simulink model "Adaptive_control_CSAD_model"  (R2017a)
settings: Solver=ode4  StartTime=0.0  StopTime=t_sim  FixedStep=0.01  RelTol=1e-3
values from neighbouring files (symbols this model uses):
  controller = 1    [Run4corner.m]
  eta_initial = [5; -1; 0]    [Run4corner.m]    (also in Simulation_plot.m = [-4; -2; 0.6*pi])
  gamma = 1.5    [Run4corner.m]
  mrs_select = 0    [Run4corner.m]
  nu_initial = [0; 0; 0]    [Run4corner.m]    (also in Simulation_plot.m)
  rho = 0.8    [Run4corner.m]
  sigma = 2    [Run4corner.m]
undefined symbols (not defined in the file or in its folder): fdesignblkfcn, gcbh
libraries: simulink x4, dsparch4 x1
(part 2 of 2)

== matlab function Adaptive_control_CSAD_model/L1 Cascade/Velocity Controller ==
  data: tau input; eta input; Alpha_DWC input; Alpha_DWC_dot input; Tau_c output; w_delta_hat_dot output; Nu input; model input; eta_hat_dot output; nu_hat_dot output; w_delta_hat input; eta_hat input; nu_hat input
function [Tau_c,w_delta_hat_dot,eta_hat_dot,nu_hat_dot]= VelocityControl(tau,eta,Alpha_DWC, Alpha_DWC_dot,Nu,model,w_delta_hat,eta_hat,nu_hat)

M = model(1:3,1:3);
C = model(1:3,4:6);
D = model(1:3,7:9);

z2 = Nu - Alpha_DWC;
psi=eta(3);
Gamma2 = diag([0.2,0.2 , 0.1745])*M;
delta_v = 0.7;
delta_r = 1;

z2_v = [z2(1), z2(2)]';
z2_r = z2(3);

first = 1/(sqrt(z2_v'*z2_v + delta_v^2));
second = 1/(sqrt(z2_r^2 + delta_r^2));

K2 = Gamma2*[first*eye(2,2) zeros(2,1); zeros(1,2) second];

z2 = Nu - Alpha_DWC;


R_T = [cos(psi) -sin(psi) 0;
       sin(psi) cos(psi) 0;
       0 0 1]';
eta_tilde = eta_hat - eta;
nu_tilde = nu_hat - Nu;


gamma_w_delta = (20*pi)^2/4; 
L1 = eye(3)*(2*pi)^2;
L2 = eye(3)*2*1.2*2*pi*3;

eta_hat_dot = -L1*eta_tilde + R_T'*Nu;
nu_hat_dot = -L2*nu_tilde + M\(tau+w_delta_hat-C*Nu-D*Nu);

w_delta_hat_dot=-gamma_w_delta*nu_tilde;

%linear model
Tau_c = M * Alpha_DWC_dot + C*Alpha_DWC+ D * Alpha_DWC - K2 * z2 -w_delta_hat;


end

== matlab function Adaptive_control_CSAD_model/L1 Cascade/ Pose Controller ==
  data: Eta_t input; Eta_tdot input; Eta_tddot input; Eta input; Nu input; Alpha output; Alphadot output
function [ Alpha ,Alphadot]  = PoseControl(Eta_t, Eta_tdot,Eta_tddot, Eta, Nu)
Gamma1 =  diag([0.08, 0.08, 0.0697]);
delta_psi = 0.5;
delta_p = 0.5;

psi = Eta(3);
r = Nu(3);

S = [0 -r  0; r  0  0; 0  0  0];
S_T = S';
R = [cos(psi) -sin(psi) 0; sin(psi) cos(psi) 0; 0 0 1];
R_T = R';

z1 = R_T * (Eta - Eta_t);

z1_p = [z1(1), z1(2)]';
z1_psi = z1(3);

first = 1/(sqrt(z1_p'*z1_p + delta_p^2));
second = 1/(sqrt(z1_psi^2 + delta_psi^2));

K1 = Gamma1*[first*eye(2,2) zeros(2,1); zeros(1,2) second];

Nu_d = R_T * Eta_tdot - K1 * z1;
Alpha = Nu_d;
z2 = Nu - Alpha;

z1dot = S_T * z1 - K1 * z1 + z2;

z1_p = [z1(1), z1(2)]';
z1_psi = z1(3);
z1_pdot = [z1dot(1), z1dot(2)]';
z1_psidot = z1dot(3);

first2 = (z1_p'*z1_pdot)/((z1_p'*z1_p + delta_p^2)^(3/2));

second2 = (z1_psi*z1_psidot)/((z1_psi^2 + delta_psi^2)^(3/2));

K1dot = - Gamma1*[first2*eye(2,2) zeros(2,1); zeros(1,2) second2];

Alphadot = R_T * Eta_tddot + S_T * R_T * Eta_tdot - K1dot * z1 - K1*z1dot;

end

== matlab function Adaptive_control_CSAD_model/Immersion and Invariance/ Pose Controller ==
  data: tau input; Eta_t input; Eta_tdot input; Eta_tddot input; Eta input; Nu input; model input; tau output; phi_dot_hat output; phi_hat input
function [tau,phi_dot_hat]  = Immersion(tau,Eta_t, Eta_tdot,Eta_tddot, Eta, Nu,model,phi_hat)

M = model(1:3,1:3);
C = model(1:3,4:6);
D = model(1:3,7:9);

Gamma1 =  diag([0.08, 0.08, 0.0697]);
delta_psi = 0.5;
delta_p = 0.5;

psi = Eta(3);
r = Nu(3);

S = [0 -r  0; r  0  0; 0  0  0];
S_T = S';
R = [cos(psi) -sin(psi) 0; sin(psi) cos(psi) 0; 0 0 1];
R_T = R';

z1 = R_T * (Eta - Eta_t);

z1_p = [z1(1), z1(2)]';
z1_psi = z1(3);

first = 1/(sqrt(z1_p'*z1_p + delta_p^2));
second = 1/(sqrt(z1_psi^2 + delta_psi^2));

K1 = Gamma1*[first*eye(2,2) zeros(2,1); zeros(1,2) second];

Nu_d = R_T * Eta_tdot - K1 * z1;
Alpha = Nu_d;
z2 = Nu - Alpha;

z1dot = S_T * z1 - K1 * z1 + z2;

z1_p = [z1(1), z1(2)]';
z1_psi = z1(3);
z1_pdot = [z1dot(1), z1dot(2)]';
z1_psidot = z1dot(3);

first2 = (z1_p'*z1_pdot)/((z1_p'*z1_p + delta_p^2)^(3/2));

second2 = (z1_psi*z1_psidot)/((z1_psi^2 + delta_psi^2)^(3/2));

K1dot = - Gamma1*[first2*eye(2,2) zeros(2,1); zeros(1,2) second2];

Alphadot = R_T * Eta_tddot + S_T * R_T * Eta_tdot - K1dot * z1 - K1*z1dot;


Gamma= diag([8, 4, 8, 8, 8, 4, 8, 8,0.4,0.4,0.4]);


r = Nu(3);
v=Nu(2);

z2 = Nu - Alpha;

Gamma2 = diag([0.2,0.2 , 0.1745])*M;
delta_v = 0.7;
delta_r = 1;

z2_v = [z2(1), z2(2)]';
z2_r = z2(3);

first = 1/(sqrt(z2_v'*z2_v + delta_v^2));
second = 1/(sqrt(z2_r^2 + delta_r^2));

K2 = Gamma2*[first*eye(2,2) zeros(2,1); zeros(1,2) second];


Phi = [0 0 0 0 0 0 0 0; abs(r)*v r abs(v)*r abs(r)*r 0 0 0 0; 0 0 0 0 abs(r)*v r abs(v)*r abs(r)*r];
Phi = [Phi R_T];
phi_dot_hat = -Gamma* Phi' * ( tau- C*Nu - D*Nu  +  Phi*(phi_hat + Gamma*Phi'*z2)- M*Alphadot);

tau = M * Alphadot + C*Alpha+ D * Alpha - K2 * z2 -  Phi*(phi_hat + Gamma*Phi'*z2);

end

== matlab function Adaptive_control_CSAD_model/10HZ1/MATLAB Function ==
  data: nu input; nu_10 output; nu_current input; i input; i_out output
function [nu_10,i_out] = hz(nu,nu_current,i)

if i==0
    nu_10=nu;
    i_out=1;
elseif i==10
    nu_10=nu;
    i_out=1;
else
    nu_10=nu_current;
    i_out=i+1;
end

== matlab function Adaptive_control_CSAD_model/Immersion and Invariance/CSAD parameters ==
  data: model output; Nu input
function model = fcn(Nu)
unction model = fcn(Nu)

X_u		= -2.332;		
X_uu 	=  0;		
X_uuu	= -8.557;

Y_v		= -4.673;   
Y_vv	= - 0.3976;
Y_vvv	= -313.3;	
Y_r		= -7.25;
Y_rr	= -3.45;
Y_rrr   = 0;

N_v		= 0;		
N_vv	= -0.2088;
N_vvv = 0;

N_r		= -7.141;
N_rr	= -4.888;
N_rrr	= -0.152;

N_rv	= 0.08;	
N_vr	= 0.08;
Y_rv	= -0.805;			
Y_vr	= -0.845;

X_ud =     -3.262;
Y_vd =     -28.89;
Y_rd =     -0.525;
N_vd =     -0.157;	
N_rd =     -13.98;

Nur  = -Y_rd;
Nuv  = -(Y_vd-X_ud);
Yur  = -X_ud;

x_g     = 0.0375;
m       = 127.92;
I_z     = 61.967;

u   = Nu(1);
v   = Nu(2);
r   = Nu(3);

d_11 = - X_u - X_uu*abs(u) - X_uuu*u^2;
d_22 = - Y_v - Y_vv*abs(v) - Y_rv*abs(r) - Y_vvv*v^2;
d_23 = - Y_r - Y_rr*abs(r) - Y_vr*abs(v) - Y_rrr*r^2 - Yur*u;
d_32 = - N_v - N_vv*abs(v) - N_rv*abs(r) - N_vvv*v^2 - Nuv*u;
d_33 = - N_r - N_rr*abs(r) - N_vr*abs(v) - N_rrr*r^2 - Nur*u;

D    = [d_11  0     0
        0     d_22  d_23
        0     d_32  d_33];

CA=[0                            0          Y_vd*v+Y_rd*r;
    0                            0                -X_ud*u;
    -Y_rd*r-Y_vd*v               X_ud*u                0];

CRB=[0             0     -m*(x_g*r+v);
     0             0      m*u;
     m*(x_g*r+v) -m*u     0]; 

C=CRB+CA;

M_RB_c=[m     0      0;
        0     m      m*x_g;
        0     m*x_g  I_z];

M_A_c=[-X_ud    0      0;
         0    -Y_vd  -Y_rd;
         0    -N_vd  -N_rd];     
    
M = M_RB_c + M_A_c;
model=[M C D];

== matlab function Adaptive_control_CSAD_model/MATLAB Function1 ==
  data: eta_L1 input; eta output; eta_II input; control_select input
function eta = switch_control(eta_L1,eta_II,control_select)

switch control_select
    
    case 1
        eta = eta_L1;
    case 2
        eta = eta_II;
    
    otherwise
        eta = [0 0 0]';
end
          
    
end

== matlab function Adaptive_control_CSAD_model/MATLAB Function2 ==
  data: eta_L1 input; eta output; eta_II input; control_select input
function eta = switch_control(eta_L1,eta_II,control_select)

switch control_select
    
    case 1
        eta = eta_L1;
    case 2
        eta = eta_II;
    
    otherwise
        eta = [0 0 0]';
end
          
    
end

== matlab function Adaptive_control_CSAD_model/L1 CG/ Pose Controller ==
  data: Eta_t input; Eta_tdot input; Eta_tddot input; Eta input; Nu input; Alpha output; Alphadot output; eta_i input; eta_i_dot output
function [ Alpha ,Alphadot,eta_i_dot]  = PoseControl(Eta_t, Eta_tdot,Eta_tddot, Eta, Nu,eta_i)
Gamma1 =  diag([0.08, 0.08, 0.0697]);
delta_psi = 0.5;
delta_p = 0.5;


psi = Eta(3);
r = Nu(3);

S = [0 -r  0; r  0  0; 0  0  0];
S_T = S';
R = [cos(psi) -sin(psi) 0; sin(psi) cos(psi) 0; 0 0 1];
R_T = R';
Eta_dot = R*Nu;
Ka = 0.01;
Kb =0.05;

eta_i_dot = Eta_tdot-Ka*(Eta-eta_i)+Kb*(Eta_t-eta_i);
eta_i_ddot = Eta_tddot - Ka*(Eta_dot-eta_i_dot) + Kb*(Eta_tdot-eta_i_dot);




z1 = R_T * (Eta - eta_i);

z1_p = [z1(1), z1(2)]';
z1_psi = z1(3);

first = 1/(sqrt(z1_p'*z1_p + delta_p^2));
second = 1/(sqrt(z1_psi^2 + delta_psi^2));

K1 = Gamma1*[first*eye(2,2) zeros(2,1); zeros(1,2) second];

z0=eta_i - Eta_t;
z0_dot = eta_i_dot - Eta_tdot;
Nu_d = R_T * eta_i_dot + R_T*Ka*z0 - K1 * z1;
Alpha = Nu_d;
z2 = Nu - Alpha;

z1dot = S_T * z1 - K1 * z1 + z2;

z1_p = [z1(1), z1(2)]';
z1_psi = z1(3);
z1_pdot = [z1dot(1), z1dot(2)]';
z1_psidot = z1dot(3);

first2 = (z1_p'*z1_pdot)/((z1_p'*z1_p + delta_p^2)^(3/2));

second2 = (z1_psi*z1_psidot)/((z1_psi^2 + delta_psi^2)^(3/2));

K1dot = - Gamma1*[first2*eye(2,2) zeros(2,1); zeros(1,2) second2];

Alphadot = R_T *eta_i_ddot + S_T * R_T * eta_i_dot +R_T*Ka*z0_dot + S_T*R_T*Ka*z0 - K1dot * z1 - K1*z1dot;

end

== matlab function Adaptive_control_CSAD_model/L1 CG/ Velocity Controller ==
  data: tau input; eta input; Alpha_DWC input; Alpha_DWC_dot input; Tau_c output; w_delta_hat_dot output; Nu input; model input; eta_hat_dot output; nu_hat_dot output; w_delta_hat input; eta_hat input; nu_hat input
function [Tau_c,w_delta_hat_dot,eta_hat_dot,nu_hat_dot]= VelocityControl(tau,eta,Alpha_DWC, Alpha_DWC_dot,Nu,model,w_delta_hat,eta_hat,nu_hat)

M = model(1:3,1:3);
C = model(1:3,4:6);
D = model(1:3,7:9);

z2 = Nu - Alpha_DWC;
psi=eta(3);
Gamma2 = diag([0.2,0.2 , 0.1745])*M;
delta_v = 0.7;
delta_r = 1;

z2_v = [z2(1), z2(2)]';
z2_r = z2(3);

first = 1/(sqrt(z2_v'*z2_v + delta_v^2));
second = 1/(sqrt(z2_r^2 + delta_r^2));

K2 = Gamma2*[first*eye(2,2) zeros(2,1); zeros(1,2) second];

z2 = Nu - Alpha_DWC;


R_T = [cos(psi) -sin(psi) 0;
       sin(psi) cos(psi) 0;
       0 0 1]';
eta_tilde = eta_hat - eta;
nu_tilde = nu_hat - Nu;


gamma_w_delta = (20*pi)^2/4; 
L1 = eye(3)*(2*pi)^2;%*2*K1;
L2 = eye(3)*2*1.2*2*pi*3;%100;%*2*K2;

eta_hat_dot = -L1*eta_tilde + R_T'*Nu;
nu_hat_dot = -L2*nu_tilde + M\(tau+w_delta_hat-C*Nu-D*Nu);

w_delta_hat_dot=-gamma_w_delta*nu_tilde;

%linear model
Tau_c = M * Alpha_DWC_dot + C*Alpha_DWC+ D * Alpha_DWC - K2 * z2 -w_delta_hat;


end

== matlab function Adaptive_control_CSAD_model/L1 CG/CSAD parameters ==
  data: model output; Nu input
function model = fcn(Nu)

X_u		= -5.35;		
X_uu 	=  0;		
X_uuu	= -19.6312;

Y_v		= -10.16;   
Y_vv	= -0.8647;
Y_vvv	= -681.1745;	

Y_r		= -7.25;
Y_rr	= -3.45;
Y_rrr   = 0;

N_v		= 0;		
N_vv	= -0.2088;
N_vvv = 0;

N_r		= -14.55;
N_rr	= -9.9597;
N_rrr	= -0.3101;

N_rv	= 0.08;	
N_vr	= 0.08;
Y_rv	= -0.805;			
Y_vr	= -0.845;

X_ud =     -10;
Y_vd =     -105;
Y_rd =     -0.525;
N_vd =     -0.157;	
N_rd =     -3.4950;

Nur  = -Y_rd;
Nuv  = -(Y_vd-X_ud);
Yur  = -X_ud;

x_g     = 0.0375;
m       = 127.92;
I_z     = 61.967;

u   = Nu(1);
v   = Nu(2);
r   = Nu(3);

d_11 = - X_u - X_uu*abs(u) - X_uuu*u^2;
d_22 = - Y_v - Y_vv*abs(v) - Y_rv*abs(r) - Y_vvv*v^2;
d_23 = - Y_r - Y_rr*abs(r) - Y_vr*abs(v) - Y_rrr*r^2 - Yur*u;
d_32 = - N_v - N_vv*abs(v) - N_rv*abs(r) - N_vvv*v^2 - Nuv*u;
d_33 = - N_r - N_rr*abs(r) - N_vr*abs(v) - N_rrr*r^2 - Nur*u;

D    = [d_11  0     0
        0     d_22  d_23
        0     d_32  d_33];

CA=[0                            0          Y_vd*v+Y_rd*r;
    0                            0                -X_ud*u;
    -Y_rd*r-Y_vd*v               X_ud*u                0];

CRB=[0             0     -m*(x_g*r+v);
     0             0      m*u;
     m*(x_g*r+v) -m*u     0]; 

C=CRB+CA;

M_RB_c=[m     0      0;
        0     m      m*x_g;
        0     m*x_g  I_z];

M_A_c=[-X_ud    0      0;
         0    -Y_vd  -Y_rd;
         0    -N_vd  -N_rd];     
    
M = M_RB_c + M_A_c;

model=[M C D];

== matlab function Adaptive_control_CSAD_model/L1 Cascade/10HZ1/MATLAB Function ==
  data: nu input; nu_10 output; nu_current input; i input; i_out output
function [nu_10,i_out] = hz(nu,nu_current,i)

if i==0
    nu_10=nu;
    i_out=1;
elseif i==10
    nu_10=nu;
    i_out=1;
else
    nu_10=nu_current;
    i_out=i+1;
end

== matlab function Adaptive_control_CSAD_model/Performance Metrics /e2 ==
  data: e1 output; eta input; eta_t input
function e1 = fcn(eta,eta_t)

x = eta(1);
y = eta(2);
psi = eta(3);

x_t = eta_t(1);
y_t = eta_t(2);
psi_t = eta_t(3);

x_tilde = x-x_t;
y_tilde = y-y_t;
psi_tilde = psi-psi_t;

e1 = sqrt((x_tilde^2)/4 + (y_tilde^2)/4 + (psi_tilde^2)/(pi/2));

== matlab function Adaptive_control_CSAD_model/L1 Cascade/10HZ4/MATLAB Function ==
  data: nu input; nu_10 output; nu_current input; i input; i_out output
function [nu_10,i_out] = hz(nu,nu_current,i)

if i==0
    nu_10=nu;
    i_out=1;
elseif i==10
    nu_10=nu;
    i_out=1;
else
    nu_10=nu_current;
    i_out=i+1;
end

== matlab function Adaptive_control_CSAD_model/Immersion and Invariance/CSAD parameters1 ==
  data: model output; Nu input
function model = fcn(Nu)

X_u		= -5.35;		
X_uu 	=  0;		
X_uuu	= -19.6312;

Y_v		= -10.16;   
Y_vv	= -0.8647;
Y_vvv	= -681.1745;	

Y_r		= -7.25;
Y_rr	= -3.45;
Y_rrr   = 0;

N_v		= 0;		
N_vv	= -0.2088;
N_vvv = 0;

N_r		= -14.55;
N_rr	= -9.9597;
N_rrr	= -0.3101;

N_rv	= 0.08;	
N_vr	= 0.08;
Y_rv	= -0.805;			
Y_vr	= -0.845;

X_ud =     -10;
Y_vd =     -105;
Y_rd =     -0.525;
N_vd =     -0.157;	
N_rd =     -3.4950;

Nur  = -Y_rd;
Nuv  = -(Y_vd-X_ud);
Yur  = -X_ud;

x_g     = 0.0375;
m       = 127.92;
I_z     = 61.967;

u   = Nu(1);
v   = Nu(2);
r   = Nu(3);

d_11 = - X_u - X_uu*abs(u) - X_uuu*u^2;
d_22 = - Y_v - Y_vv*abs(v) - Y_rv*abs(r) - Y_vvv*v^2;
d_23 = - Y_r - Y_rr*abs(r) - Y_vr*abs(v) - Y_rrr*r^2 - Yur*u;
d_32 = - N_v - N_vv*abs(v) - N_rv*abs(r) - N_vvv*v^2 - Nuv*u;
d_33 = - N_r - N_rr*abs(r) - N_vr*abs(v) - N_rrr*r^2 - Nur*u;

D    = [d_11  0     0
        0     d_22  d_23
        0     d_32  d_33];

CA=[0                            0          Y_vd*v+Y_rd*r;
    0                            0                -X_ud*u;
    -Y_rd*r-Y_vd*v               X_ud*u                0];

CRB=[0             0     -m*(x_g*r+v);
     0             0      m*u;
     m*(x_g*r+v) -m*u     0]; 

C=CRB+CA;

M_RB_c=[m     0      0;
        0     m      m*x_g;
        0     m*x_g  I_z];

M_A_c=[-X_ud    0      0;
         0    -Y_vd  -Y_rd;
         0    -N_vd  -N_rd];     
    
M = M_RB_c + M_A_c;

model=[M C D];

== matlab function Adaptive_control_CSAD_model/Performance Metrics /e3 ==
  data: tau_dot output; tau_dot_in input
function tau_dot = fcn(tau_dot_in)

tau1 = tau_dot_in(1);
tau2 = tau_dot_in(2);
tau3 = tau_dot_in(3);



tau_dot = sqrt((tau1^2) + (tau2^2) + (tau3^2));

== matlab function Adaptive_control_CSAD_model/L1 CG/10HZ1/MATLAB Function ==
  data: nu input; nu_10 output; nu_current input; i input; i_out output
function [nu_10,i_out] = hz(nu,nu_current,i)

if i==0
    nu_10=nu;
    i_out=1;
elseif i==10
    nu_10=nu;
    i_out=1;
else
    nu_10=nu_current;
    i_out=i+1;
end

== matlab function Adaptive_control_CSAD_model/Performance Metrics /|P|1 ==
  data: nu input; P output; tau input
function P  = fcn(nu, tau)
P = abs(nu'*tau);

== matlab function Adaptive_control_CSAD_model/Immersion and Invariance/ Pose Controller1 ==
  data: tau input; Eta_t input; Eta_t_dot input; Eta_t_ddot input; Eta input; Nu input; model input; tau output; phi_dot_hat output; phi_hat input
function [tau,phi_dot_hat]  = Immersion(tau,Eta_t, Eta_t_dot,Eta_t_ddot, Eta, Nu,model,phi_hat)

M = model(1:3,1:3);
C = model(1:3,4:6);
D = model(1:3,7:9);



K1 = diag([0.08 0.08 0.0698]);
K2 = diag( [0.2 0.2 0.174]*M);%diag([5, 7, 15]);

Gamma= diag([8, 4, 8, 8, 8, 4, 8, 8,0.4,0.4,0.4]);

psi = Eta(3);
r = Nu(3);
v=Nu(2);

S = [0 -r  0; r  0  0; 0  0  0];
S_T = S';
R = [cos(psi) -sin(psi) 0; sin(psi) cos(psi) 0; 0 0 1];
R_T = R';


z_1 = R_T*(Eta-Eta_t);


alpha = R_T*Eta_t_dot - K1*z_1;

z_2 = Nu - alpha;
z_1_dot = S_T * z_1 - K1 * z_1 + z_2;
alpha_dot = R_T*Eta_t_ddot + S_T*R_T*Eta_t_dot - K1*z_1_dot;

Phi = [0 0 0 0 0 0 0 0; abs(r)*v r abs(v)*r abs(r)*r 0 0 0 0; 0 0 0 0 abs(r)*v r abs(v)*r abs(r)*r];
Phi = [Phi R_T];
phi_dot_hat = -Gamma* Phi' * ( tau- C*Nu - D*Nu  +  Phi*(phi_hat + Gamma*Phi'*z_2)- M*alpha_dot);

tau = -K2*z_2 - z_1 + C*Nu - D*Nu  +  Phi*(phi_hat + Gamma*Phi'*z_2)- M*alpha_dot;

end

== matlab function Adaptive_control_CSAD_model/Satutation/MATLAB Function1 ==
  data: tau input; tau_out output; tau_mrs input; mrs input
function tau_out = switch_control(tau,tau_mrs,mrs)

switch mrs
    
    case 0
        tau_out = tau;
    case 1
        tau_out = tau_mrs;
    
    otherwise
        tau_out = [0 0 0]';
end
          
    
end

== matlab function Adaptive_control_CSAD_model/Satutation1/MATLAB Function1 ==
  data: tau input; tau_out output; tau_mrs input; mrs input
function tau_out = switch_control(tau,tau_mrs,mrs)

switch mrs
    
    case 0
        tau_out = tau;
    case 1
        tau_out = tau_mrs;
    
    otherwise
        tau_out = [0 0 0]';
end
          
    
end

== matlab function Adaptive_control_CSAD_model/Satutation1/MRS 1/Magnitude Constraints2 ==
  data: delta input; Tau_mrs output
function Tau_mrs = MagConstr(delta)


%mag_constr = [2.88;1.60;1.36]; %for lab (same ratio, but lower)
mag_constr = [5;5;3];
Tau_mrs = [0;0;0];

for n = 1:length(delta)
    
    if delta(n) <= -mag_constr(n)
        Tau_mrs(n) = -mag_constr(n);
    end
    
    if ((delta(n) > -mag_constr(n)) && (delta(n) < mag_constr(n)))
        Tau_mrs(n) = delta(n);
    end
    
    if delta(n) >= mag_constr(n)
        Tau_mrs(n) = mag_constr(n);
    end
    
end
    
end

== matlab function Adaptive_control_CSAD_model/Satutation1/MRS 1/Rate Constraints1 ==
  data: epsilon input; delta_dot output
function delta_dot = RateConstr(epsilon)

rate_constr = [2.88;1.60;1.36]*1.2; %N


delta_dot = [0;0;0];

for n = 1:length(epsilon)
    
    if epsilon(n) <= -rate_constr(n)
        delta_dot(n) = -rate_constr(n);
    end
    
    if ((epsilon(n) > -rate_constr(n)) && (epsilon(n) < rate_constr(n)))
        delta_dot(n) = epsilon(n);
    end
    
    if epsilon(n) >= rate_constr(n)
        delta_dot(n) = rate_constr(n);
    end
    
end
    
end

== matlab function Adaptive_control_CSAD_model/Satutation/MRS 2/Magnitude Constraints2 ==
  data: delta input; Tau_mrs output
function Tau_mrs = MagConstr(delta)


%mag_constr = [2.88;1.60;1.36]; %for lab (same ratio, but lower)
mag_constr =  [5, 5, 3];
Tau_mrs = [0;0;0];

for n = 1:length(delta)
    
    if delta(n) <= -mag_constr(n)
        Tau_mrs(n) = -mag_constr(n);
    end
    
    if ((delta(n) > -mag_constr(n)) && (delta(n) < mag_constr(n)))
        Tau_mrs(n) = delta(n);
    end
    
    if delta(n) >= mag_constr(n)
        Tau_mrs(n) = mag_constr(n);
    end
    
end
    
end

== matlab function Adaptive_control_CSAD_model/Satutation/MRS 2/Rate Constraints1 ==
  data: epsilon input; delta_dot output
function delta_dot = RateConstr(epsilon)

rate_constr =  [2.88, 1.60, 1.36]; %N


delta_dot = [0;0;0];

for n = 1:length(epsilon)
    
    if epsilon(n) <= -rate_constr(n)
        delta_dot(n) = -rate_constr(n);
    end
    
    if ((epsilon(n) > -rate_constr(n)) && (epsilon(n) < rate_constr(n)))
        delta_dot(n) = epsilon(n);
    end
    
    if epsilon(n) >= rate_constr(n)
        delta_dot(n) = rate_constr(n);
    end
    
end
    
end

== matlab function Adaptive_control_CSAD_model/CSAD Vessel2/MATLAB Function2 ==
  data: eta input; tau_s input; Eta_dot output; Nu input; Nu_dot output; gamma input; sigma input; rho input
function [Eta_dot,Nu_dot] = Vessel(eta,tau_s,Nu,gamma,sigma,rho)

Nu_dot = CSAD_full(Nu,tau_s,gamma,sigma,rho);

yaw = eta(3);

R =[cos(yaw) -sin(yaw) 0;
            sin(yaw)  cos(yaw) 0;
            0         0        1]; 
Eta_dot = R*Nu;
end

== matlab function Adaptive_control_CSAD_model/10HZ4/MATLAB Function ==
  data: nu input; nu_10 output; nu_current input; i input; i_out output
function [nu_10,i_out] = hz(nu,nu_current,i)

if i==0
    nu_10=nu;
    i_out=1;
elseif i==10
    nu_10=nu;
    i_out=1;
else
    nu_10=nu_current;
    i_out=i+1;
end

== matlab function Adaptive_control_CSAD_model/10HZ3/MATLAB Function ==
  data: nu input; nu_10 output; nu_current input; i input; i_out output
function [nu_10,i_out] = hz(nu,nu_current,i)

if i==0
    nu_10=nu;
    i_out=1;
elseif i==10
    nu_10=nu;
    i_out=1;
else
    nu_10=nu_current;
    i_out=i+1;
end

== matlab function Adaptive_control_CSAD_model/10HZ2/MATLAB Function ==
  data: nu input; nu_10 output; nu_current input; i input; i_out output
function [nu_10,i_out] = hz(nu,nu_current,i)

if i==0
    nu_10=nu;
    i_out=1;
elseif i==10
    nu_10=nu;
    i_out=1;
else
    nu_10=nu_current;
    i_out=i+1;
end

== matlab function Adaptive_control_CSAD_model/10HZ5/MATLAB Function ==
  data: nu input; nu_10 output; nu_current input; i input; i_out output
function [nu_10,i_out] = hz(nu,nu_current,i)

if i==0
    nu_10=nu;
    i_out=1;
elseif i==10
    nu_10=nu;
    i_out=1;
else
    nu_10=nu_current;
    i_out=i+1;
end

== matlab function Adaptive_control_CSAD_model/10HZ6/MATLAB Function ==
  data: nu input; nu_10 output; nu_current input; i input; i_out output
function [nu_10,i_out] = hz(nu,nu_current,i)

if i==0
    nu_10=nu;
    i_out=1;
elseif i==10
    nu_10=nu;
    i_out=1;
else
    nu_10=nu_current;
    i_out=i+1;
end

== matlab function Adaptive_control_CSAD_model/CSAD Vessel/MATLAB Function1 ==
  data: eta input; tau_s input; Eta_dot output; Nu input; Nu_dot output; gamma input; sigma input; rho input
function [Eta_dot,Nu_dot] = Vessel(eta,tau_s,Nu,gamma,sigma,rho)

Nu_dot = CSAD_full(Nu,tau_s,gamma,sigma,rho);

yaw = eta(3);

R =[cos(yaw) -sin(yaw) 0;
            sin(yaw)  cos(yaw) 0;
            0         0        1]; 
Eta_dot = R*Nu;
end

== matlab function Adaptive_control_CSAD_model/Satutation3/MATLAB Function1 ==
  data: tau input; tau_out output; tau_mrs input; mrs input
function tau_out = switch_control(tau,tau_mrs,mrs)

switch mrs
    
    case 0
        tau_out = tau;
    case 1
        tau_out = tau_mrs;
    
    otherwise
        tau_out = [0 0 0]';
end
          
    
end

== matlab function Adaptive_control_CSAD_model/Satutation3/MRS 2/Magnitude Constraints2 ==
  data: delta input; Tau_mrs output
function Tau_mrs = MagConstr(delta)


%mag_constr = [2.88;1.60;1.36]; %for lab (same ratio, but lower)
mag_constr =  [5, 5, 3];
Tau_mrs = [0;0;0];

for n = 1:length(delta)
    
    if delta(n) <= -mag_constr(n)
        Tau_mrs(n) = -mag_constr(n);
    end
    
    if ((delta(n) > -mag_constr(n)) && (delta(n) < mag_constr(n)))
        Tau_mrs(n) = delta(n);
    end
    
    if delta(n) >= mag_constr(n)
        Tau_mrs(n) = mag_constr(n);
    end
    
end
    
end

== matlab function Adaptive_control_CSAD_model/Satutation3/MRS 2/Rate Constraints1 ==
  data: epsilon input; delta_dot output
function delta_dot = RateConstr(epsilon)

rate_constr =  [2.88, 1.60, 1.36]; %N


delta_dot = [0;0;0];

for n = 1:length(epsilon)
    
    if epsilon(n) <= -rate_constr(n)
        delta_dot(n) = -rate_constr(n);
    end
    
    if ((epsilon(n) > -rate_constr(n)) && (epsilon(n) < rate_constr(n)))
        delta_dot(n) = epsilon(n);
    end
    
    if epsilon(n) >= rate_constr(n)
        delta_dot(n) = rate_constr(n);
    end
    
end
    
end

== matlab function Adaptive_control_CSAD_model/MATLAB Function ==
  data: eta_L1 input; eta output; eta_II input; control_select input
function eta = switch_control(eta_L1,eta_II,control_select)

switch control_select
    
    case 1
        eta = eta_L1;
    case 2
        eta = eta_II;
    
    otherwise
        eta = [0 0 0]';
end
          
    
end

== matlab function Adaptive_control_CSAD_model/Magnitude Constraints2 ==
  data: Tau_c input; Tau_s output
function Tau_s = MagConstr(Tau_c)

mag_constr = [1.1089, 0.6387, 0.6176]; %real
% mag_constr = [1, 0.58, 0.56]; %for lab (same ratio, but lower)

Tau_s = [0;0;0];

for n = 1:length(Tau_c)
    
    if Tau_c(n) <= -mag_constr(n)
        Tau_s(n) = -mag_constr(n);
    end
    
    if ((Tau_c(n) > -mag_constr(n)) && (Tau_c(n) < mag_constr(n)))
        Tau_s(n) = Tau_c(n);
    end
    
    if Tau_c(n) >= mag_constr(n)
        Tau_s(n) = mag_constr(n);
    end
    
end
    
end
